simulink model "model2_fixed"  (R2015a)
settings: Solver=ode3  StartTime=0.0  StopTime=10.0  FixedStep=0.001  RelTol=1e-3
values from neighbouring files (symbols this model uses):
  th0 = 1    [starter2.m]
  x0 = 1    [starter2.m]
  z0 = 1    [starter2.m]
settings Model: Creator=zanez  LastModifiedBy=Subodh

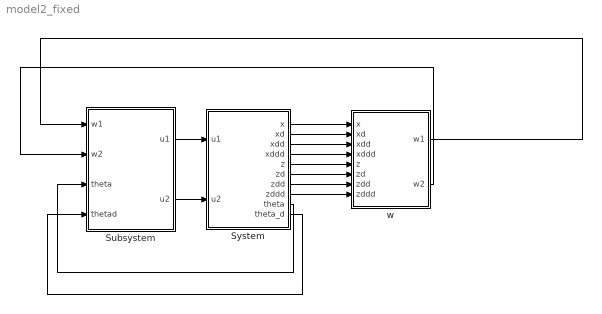
== system model2_fixed ==
  Subsystem : Subsystem
  System : Subsystem
  w : Subsystem
  wires:
  Subsystem/2(u2) -> System/2(u2)
  Subsystem/1(u1) -> System/1(u1)
  w/1(w1) -> Subsystem/1(w1)
  w/2(w2) -> Subsystem/2(w2)
  System/9(theta) -> Subsystem/3(theta)
  System/10(theta_d) -> Subsystem/4(thetad)
  System/1(x) -> w/1(x)
  System/2(xd) -> w/2(xd)
  System/3(xdd) -> w/3(xdd)
  System/4(xddd) -> w/4(xddd)
  System/5(z) -> w/5(z)
  System/6(zd) -> w/6(zd)
  System/7(zdd) -> w/7(zdd)
  System/8(zddd) -> w/8(zddd)

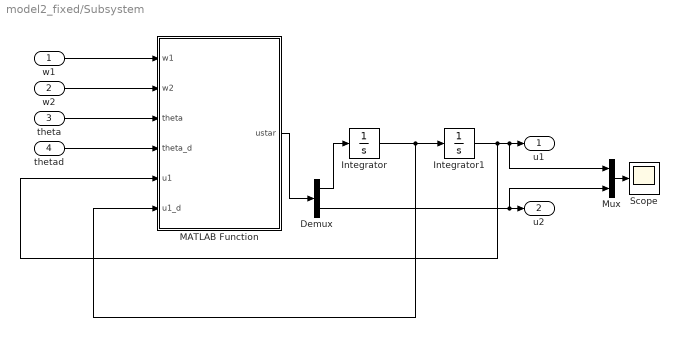
== system model2_fixed/Subsystem ==
  w1 : Inport
  w2 : Inport  Port=2
  theta : Inport  Port=3
  thetad : Inport  Port=4
  Demux : Demux  Outputs=2
  Integrator : Integrator
  Integrator1 : Integrator  InitialCondition=1
  MATLAB Function : MATLAB Function  TreatAsAtomicUnit=on
      settings: PermitHierarchicalResolution=ParametersOnly
  Mux : Mux  Inputs=2
  Scope : Scope
      settings: TimeRange=auto  MaxDataPoints=5000  SaveToWorkspace=off  SaveName=ScopeData  YMin=-522.12281  YMax=877.33327  SampleTime=-1  DataFormat=Array
  u1 : Outport
  u2 : Outport  Port=2
  wires:
  theta/1 -> MATLAB Function/3(theta)
  Demux/2 -> Mux/2, u2/1
  MATLAB Function/1(ustar) -> Demux/1
  w1/1 -> MATLAB Function/1(w1)
  w2/1 -> MATLAB Function/2(w2)
  Demux/1 -> Integrator/1
  Integrator/1 -> MATLAB Function/6(u1_d), Integrator1/1
  Integrator1/1 -> MATLAB Function/5(u1), Mux/1, u1/1
  thetad/1 -> MATLAB Function/4(theta_d)
  Mux/1 -> Scope/1

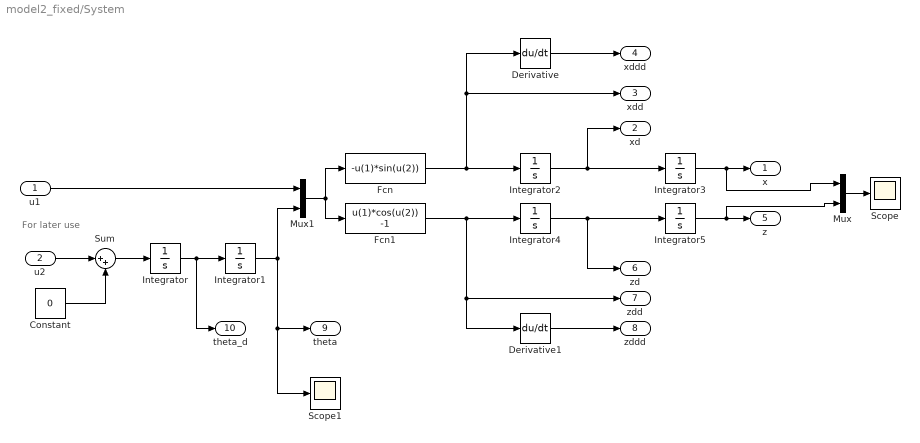
== system model2_fixed/System ==
  note: For later use
  u1 : Inport
  u2 : Inport  Port=2
  Constant : Constant  Value=0
  Derivative : Derivative
  Derivative1 : Derivative
  Fcn : Fcn  Expr=-u(1)*sin(u(2))
  Fcn1 : Fcn  Expr=u(1)*cos(u(2)) -1
  Integrator : Integrator
  Integrator1 : Integrator  InitialCondition=th0
  Integrator2 : Integrator
  Integrator3 : Integrator  InitialCondition=x0
  Integrator4 : Integrator
  Integrator5 : Integrator  InitialCondition=z0
  Mux : Mux  Inputs=2
  Mux1 : Mux  Inputs=2
  Scope : Scope
      settings: TimeRange=auto  LimitDataPoints=on  MaxDataPoints=5000  SaveToWorkspace=off  YMin=-10  YMax=10  SampleTime=-1  DataFormat=Array
  Scope1 : Scope
      settings: TimeRange=auto  LimitDataPoints=on  MaxDataPoints=5000  SaveToWorkspace=off  SaveName=ScopeData2  YMin=-10  YMax=10  SampleTime=-1  DataFormat=Array
  Sum : Sum  Inputs=|++
  x : Outport
  xd : Outport  Port=2
  xdd : Outport  Port=3
  xddd : Outport  Port=4
  z : Outport  Port=5
  zd : Outport  Port=6
  zdd : Outport  Port=7
  zddd : Outport  Port=8
  theta : Outport  Port=9
  theta_d : Outport  Port=10
  wires:
  u1/1 -> Mux1/1
  u2/1 -> Sum/1
  Constant/1 -> Sum/2
  Integrator/1 -> Integrator1/1, theta_d/1
  Sum/1 -> Integrator/1
  Integrator1/1 -> Mux1/2, theta/1, Scope1/1
  Fcn/1 -> xdd/1, Derivative/1, Integrator2/1
  Integrator2/1 -> Integrator3/1, xd/1
  Derivative/1 -> xddd/1
  Integrator3/1 -> Mux/1, x/1
  Fcn1/1 -> zdd/1, Derivative1/1, Integrator4/1
  Integrator4/1 -> zd/1, Integrator5/1
  Derivative1/1 -> zddd/1
  Integrator5/1 -> Mux/2, z/1
  Mux/1 -> Scope/1
  Mux1/1 -> Fcn/1, Fcn1/1

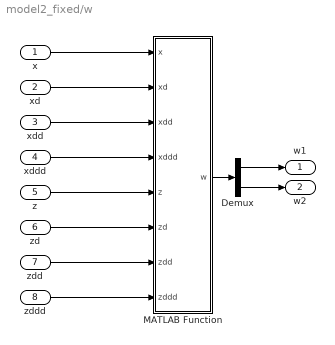
== system model2_fixed/w ==
  x : Inport
  xd : Inport  Port=2
  xdd : Inport  Port=3
  xddd : Inport  Port=4
  z : Inport  Port=5
  zd : Inport  Port=6
  zdd : Inport  Port=7
  zddd : Inport  Port=8
  Demux : Demux  Outputs=2
  MATLAB Function : MATLAB Function  TreatAsAtomicUnit=on
      settings: PermitHierarchicalResolution=ParametersOnly
  w1 : Outport
  w2 : Outport  Port=2
  wires:
  xd/1 -> MATLAB Function/2(xd)
  x/1 -> MATLAB Function/1(x)
  zd/1 -> MATLAB Function/6(zd)
  z/1 -> MATLAB Function/5(z)
  MATLAB Function/1(w) -> Demux/1
  Demux/1 -> w1/1
  Demux/2 -> w2/1
  xdd/1 -> MATLAB Function/3(xdd)
  zdd/1 -> MATLAB Function/7(zdd)
  zddd/1 -> MATLAB Function/8(zddd)
  xddd/1 -> MATLAB Function/4(xddd)

== matlab function model2_fixed/Subsystem/MATLAB Function ==
  data: ustar output; w1 input; w2 input; theta input; theta_d input; u1 input; u1_d input
function ustar = fcn(w1,w2, theta, theta_d, u1,u1_d)
%#codegen
% th = theta;
% bstarI = [    -sin(th),     cos(th); -cos(th)/u1, -sin(th)/u1];
% w1ma = w1 + 2*u1*cos(th)*thd+u1*sin(th)*thd^2;
% w2ma = w2 + u1*cos(th)*thd^2+2*u1*sin(th)*thd;

a_s = [-2*u1_d*theta_d*cos(theta) + u1*(theta_d)^2*sin(theta);...
              -2*u1_d*theta_d*sin(theta) - u1*(theta_d)^2*cos(theta)];

b_s = [-sin(theta) -u1*cos(theta); cos(theta) -u1*sin(theta)];
w = [w1;w2];
ustar = inv(b_s)*(w-a_s);
% ustar = bstarI*[w1ma;w2ma];

== matlab function model2_fixed/w/MATLAB Function ==
  data: x input; xd input; xdd input; xddd input; z input; w output; zd input; zdd input; zddd input
function w = fcn(x, xd, xdd, xddd, z, zd, zdd, zddd)
%#codegen
s0 = 5;
k11 = 4*s0; k12 = 6*s0^2; k13 = 4*s0^3; k14 = s0^4;
k21 = 4*s0; k22 = 6*s0^2; k23 = 4*s0^3; k24 = s0^4;
w1 = -k11*xddd-k12*xdd-k13*xd-k14*x;
w2 = -k21*zddd-k22*zdd-k23*zd-k24*z;
w = [w1;w2];
